simulink model "sampling_101"  (Simulink 7.4)
settings: Solver=ode45  StartTime=0.0  StopTime=inf  MaxStep=0.01/8000  RelTol=1e-3
libraries: dsparch4 x3, simulink x1
settings Model: Creator=Dick Benson  LastModifiedBy=Dick
settings DataIOCC: SignalLoggingName=sigsOut
settings OptimizationCC: InitFltsAndDblsToZero=on
settings DebuggingCC: SaveWithParameterizedLinksMsg=none  SignalResolutionControl=TryResolveAllWithWarning  SolverPrmCheckMsg=none  MultiTaskDSMMsg=warning  MultiTaskCondExecSysMsg=none  StrictBusMsg=None
settings HardwareCC: TargetUnknown=on
settings RTWCC: IncludeERTFirstTime=on
settings GRTTargetCC: TargetFcnLib=ansi_tfl_tmw.mat

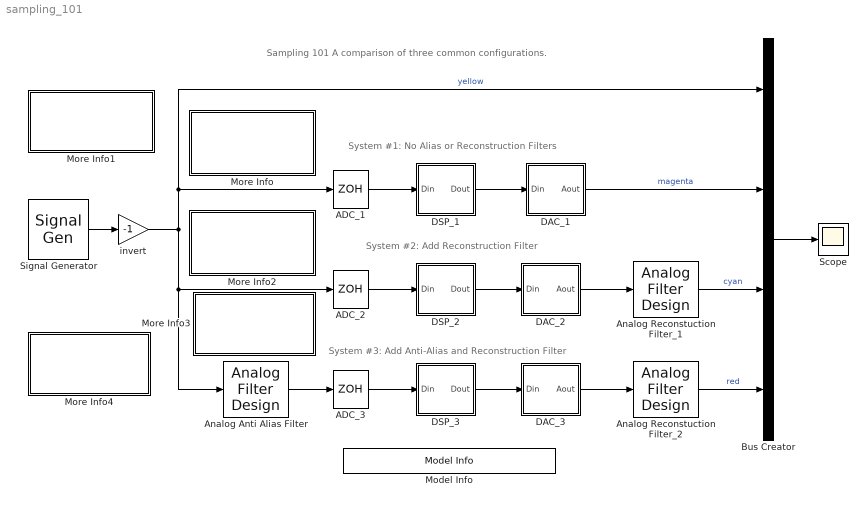
== system sampling_101 ==
  note: System #1: No Alias or Reconstruction Filters
  note: System #2: Add Reconstruction Filter
  note: System #3: Add Anti-Alias and Reconstruction Filter
  note: Sampling 101
      | A comparison of three common configurations.
  ADC_1 : ZeroOrderHold  SampleTime=1/8000
  ADC_2 : ZeroOrderHold  SampleTime=1/8000
  ADC_3 : ZeroOrderHold  SampleTime=1/8000
  Analog Anti Alias Filter : dsparch4/Analog Filter Design  method=Elliptic  filttype=Lowpass  N=8  Wlo=2*pi*8000/2.56  Whi=80  Rp=1  Rs=80
  Analog Reconstuction Filter_1 : dsparch4/Analog Filter Design  method=Elliptic  filttype=Lowpass  N=8  Wlo=2*pi*8000/2.56  Whi=80  Rp=1  Rs=80
  Analog Reconstuction Filter_2 : dsparch4/Analog Filter Design  method=Elliptic  filttype=Lowpass  N=8  Wlo=2*pi*8000/2.56  Whi=80  Rp=1  Rs=80
  Bus Creator : BusCreator
  DAC_1 : Subsystem
  DAC_2 : Subsystem
  DAC_3 : Subsystem
  DSP_1 : Subsystem
  DSP_2 : Subsystem
  DSP_3 : Subsystem
  Model Info : simulink/Model-Wide Utilities/Model Info  SystemSampleTime=-1  InitialBlockCM=None  BlockCM=None  Frame=on  DisplayStringWithTags=Copywrite 2005-2010 The MathWorks, Inc.  HorizontalTextAlignment=Center  LeftAlignmentValue=0.5  SourceBlockDiagram=sampling_101  TagMaxNumber=20
  More Info : Subsystem
      mask Display: disp('Double click for\n information on \nSystem 1')
  More Info1 : Subsystem
      mask Display: disp('Double click for\n model overview')
  More Info2 : Subsystem
      mask Display: disp('Double click for\n information on \nSystem 2')
  More Info3 : Subsystem
      mask Display: disp('Double click for\n information on \nSystem 3')
  More Info4 : Subsystem
      mask Display: disp('Double click for\n Conclusion')
  Scope : Scope
      settings: TimeRange=0.003998400639744102  YMin=-1.5  YMax=1.5
  Signal Generator : SignalGenerator  WaveForm=square  Frequency=250.1
  invert : Gain  Gain=-1  ParameterDataType=sfix(16)  ParameterScaling=2^0  OutDataType=sfix(16)  OutScaling=2^0  SaturateOnIntegerOverflow=on  OutDataTypeStr=Inherit: Same as input  ParamDataTypeStr=Inherit: Same as input
  wires:
  Signal Generator/1 -> invert/1
  ADC_1/1 -> DSP_1/1(Din)
  ADC_2/1 -> DSP_2/1(Din)
  Analog Reconstuction Filter_1/1 -> Bus Creator/3  "cyan"
  Analog Anti Alias Filter/1 -> ADC_3/1
  ADC_3/1 -> DSP_3/1(Din)
  Analog Reconstuction Filter_2/1 -> Bus Creator/4  "red"
  Bus Creator/1 -> Scope/1
  DAC_1/1(Aout) -> Bus Creator/2  "magenta"
  DAC_2/1(Aout) -> Analog Reconstuction Filter_1/1
  DAC_3/1(Aout) -> Analog Reconstuction Filter_2/1
  invert/1 -> Bus Creator/1, ADC_1/1, Analog Anti Alias Filter/1, ADC_2/1  "yellow"
  DSP_1/1(Dout) -> DAC_1/1(Din)
  DSP_2/1(Dout) -> DAC_2/1(Din)
  DSP_3/1(Dout) -> DAC_3/1(Din)

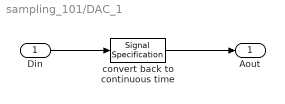
== system sampling_101/DAC_1 ==
  Din : Inport  OutDataType=sfix(16)  OutScaling=2^0
  convert back to continuous time : SignalSpecification  SampleTime=0  OutDataType=sfix(16)  OutScaling=2^0
  Aout : Outport  OutDataType=sfix(16)  OutScaling=2^0
  wires:
  convert back to continuous time/1 -> Aout/1
  Din/1 -> convert back to continuous time/1

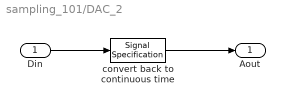
== system sampling_101/DAC_2 ==
  Din : Inport  OutDataType=sfix(16)  OutScaling=2^0
  convert back to continuous time : SignalSpecification  SampleTime=0  OutDataType=sfix(16)  OutScaling=2^0
  Aout : Outport  OutDataType=sfix(16)  OutScaling=2^0
  wires:
  Din/1 -> convert back to continuous time/1
  convert back to continuous time/1 -> Aout/1

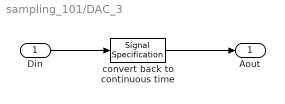
== system sampling_101/DAC_3 ==
  Din : Inport  OutDataType=sfix(16)  OutScaling=2^0
  convert back to continuous time : SignalSpecification  SampleTime=0  OutDataType=sfix(16)  OutScaling=2^0
  Aout : Outport  OutDataType=sfix(16)  OutScaling=2^0
  wires:
  convert back to continuous time/1 -> Aout/1
  Din/1 -> convert back to continuous time/1

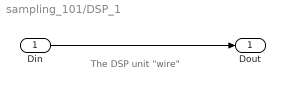
== system sampling_101/DSP_1 ==
  note: The DSP unit "wire"
  Din : Inport  OutDataType=sfix(16)  OutScaling=2^0
  Dout : Outport  OutDataType=sfix(16)  OutScaling=2^0
  wires:
  Din/1 -> Dout/1

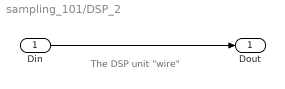
== system sampling_101/DSP_2 ==
  note: The DSP unit "wire"
  Din : Inport  OutDataType=sfix(16)  OutScaling=2^0
  Dout : Outport  OutDataType=sfix(16)  OutScaling=2^0
  wires:
  Din/1 -> Dout/1

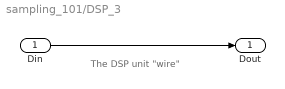
== system sampling_101/DSP_3 ==
  note: The DSP unit "wire"
  Din : Inport  OutDataType=sfix(16)  OutScaling=2^0
  Dout : Outport  OutDataType=sfix(16)  OutScaling=2^0
  wires:
  Din/1 -> Dout/1

== system sampling_101/More Info ==
  note: Sampled  Data Systems
      | (System 1)
  note: System #1 lacks continuous time filtering (bandlimiting) before the ADC and after the DAC.
      | This configuration is commonly employed in control systems applications.  The magenta  trace shows
      | that result of passing the function generator signal through a perfect ADC and DAC sampling at 8000 Hz.
      | Obviously, we have something other than a wire in the system.  The first thing one notices is the magenta signal drifts to
      | the right as the simulation runs. This is due to the fact that the square wave frequency and the sampling frequency are
      | not related in a trivial way. In other words Fs ~= k*Fsig but NOT  Fs=k*Fsig.  Change the function generator to a sine wave.
      |  One then sees the "stair steps" in the magenta trace due to the most basic form of signal reconstruction:
      | holding the sample value between sampling instants.
      |
      | Clearly, this is not a time invariant system!

== system sampling_101/More Info1 ==
  note: The objective is to demonstrate some of the effects of processing a continuous time signal by a "real world"
      | discrete time system.
      |
      | Three common sampled data system configurations are shown.  The systems are all "processing" the same
      | repetitive step input (square wave). This is shown as the yellow trace on the scope block. The repetition rate
      | of the square wave was chosen to be 250.1 Hz and the ADC sampling rate is set to 8000 Hz. Therefore, there
      | are a non-integer number of samples per cycle, as is typical in the "real world".  The scope block time axis
      | is set to be precisely one period of the input signal, and therefore the square wave display (yellow) is fixed in time
      | with respect to the scope axis. This is exactly equivalent to triggering a real oscilloscope on the function generator
      | signal that is driving the system. In all cases, the digital signal processing is reduced to its simplest form:
      |  "a virtual wire". Therefore DSP subsystem is simply there as a placeholder to explicitly show where digital
      | signal processing would occur.
      |
      | Since the DSP system is a "wire", in the ideal case, the digital system would exactly reproduce the
      | input signal at its output.  for this to happen, the input signal must be sampled by by an ADC at a rate that is
      | twice the signal bandwidth. The DAC must be followed by  a  "brick wall" reconstruction filter.
      | All of these elements must have zero delay no less!   Clearly replacing a wire with a DSP system is not possible,
      | but fortunately, not very desirable either! However, the unit wire does serve as a useful example that allows
      | one to observe the effects due to the conversion from continuous time to discrete time, and then from
      | discrete time back to continuous time.
  note: Sampled  Data Systems
      | (what they may not have told you)

== system sampling_101/More Info2 ==
  note: Leaving the source set to a sine wave for the moment, it can be seen that the output from System #2 (cyan)
      | lacks the "stair steps", AND the delay from input to output appears to be a constant as well. In other words, we have
      | made a better approximation to the wire, but a the expense of introducing a delay.  Modest delay in an audio or video  processing
      |  system is typically an acceptable tradeoff. However, it can be unacceptable in a control system where the signal
      | processing is in the feedback portion of the design. Delay introduces a phase shift that linearly increases with frequency
      | and this tends to de-stabilize the loop by lowering the loop phase margin.
      |
      | Now, change the source back to the square wave.  Two things become apparent.
      |
      | First, there is considerable overshoot  and ringing in the output. This is due to the transient response of the low pass
      | reconstruction filter. The elliptic filter used for this example has excellent frequency domain characteristics
      |  (small transition between pass-band and stop-band), but poor time domain performance.
      |
      | Try changing the filter to the Bessel and note the improvement in the time domain. However,
      | be advised, the frequency domain performance will not be as good: less alias suppression at high frequencies.
  note: Sampled  Data Systems
      | (System 2)

== system sampling_101/More Info3 ==
  note: Sampled  Data Systems
      | (System 3)
  note: Leaving the source set to the square wave, one can see output from System #3 (red), has yet more delay and more overshoot,
      | BUT, exhibits a constant delay. The response does not wander in time like systems 1&2. This system is linear time invariant.
      |
      | The reason: the input has now been bandlimited by the anti-alias filter.
      | The price: more hardware, more delay, degraded transient response.
      |
      | Try changing the first, and then both filters to the Bessel and note the marked improvement in the time domain. However,
      | as before, the frequency domain performance will not be as good: less alias and image suppression at high frequencies.

== system sampling_101/More Info4 ==
  note: The design of practical digital signal processing systems involves many tradeoffs. When used in feedback control systems,
      | the processing delay is often a critical issue.  Anti alias and Reconstruction filters (Anti Image) can move the system performance
      | closer to "ideal" at the expense of more hardware and input to output delay.  The choice between filters that have good time domain
      | properties versus those with good frequency domain properties is a sensitive function of the application. For instance, an elliptic filter
      | would be a good choice for Software Defined Radio applications because the frequency domain characteristics are typically
      | more important than the time domain.
      |
      | However, if the signal occupies a significant portion of the filter pass band (eg Video ) then the non linear phase versus frequency
      | and resulting poor transient response make filters such as the Bessel variety more attractive.  Lowpass filters were used for
      | these examples, but the results hold for the bandpass case as well.
      |
      | In the end, the design engineer must wrestle with these tradeoffs.
      |
      | The good news: Simulink does a seamless job of high fidelity simulations of these important effects.
  note: Sampled  Data Systems
      | (Conclusion)
